simulink model "SENSORES"  (R2017b)
settings: Solver=FixedStepAuto  StartTime=0.0  StopTime=4.25  FixedStep=0.01  RelTol=1e-3  EnableMultiTasking=on
libraries: arduinolib x3
settings Model: SimulationMode=external  ExtModeTrigDuration=2  Creator=ferca  LastModifiedBy=Dr. Candia
settings OptimizationCC: EnhancedBackFolding=on  PassReuseOutputArgsThreshold=0  MaxStackSize=64  OptimizeBlockOrder=speed  DifferentSizesBufferReuse=on
settings DebuggingCC: ParameterTunabilityLossMsg=error
settings HardwareCC: ProdBitPerInt=16  ProdBitPerPointer=16  ProdBitPerSizeT=16  ProdBitPerPtrDiffT=16  ProdLargestAtomicFloat=None  ProdWordSize=8  ProdHWDeviceType=Atmel->AVR
settings SFSimCC: SimUseLocalCustomCode=on  MATLABDynamicMemAlloc=off
settings RTWCC: SystemTargetFile=ert.tlc  HardwareBoard=Arduino Uno  TLCOptions=-aInlineSetEventsForThisBaseRateFcn=TLC_FALSE -aSuppressMultiTaskScheduler=TLC_FALSE -aRateBasedStepFcn=1  TemplateMakefile=ert_default_tmf  GenerateReport=on  RTWUseLocalCustomCode=on  Toolchain=Arduino AVR  BuildConfiguration=Faster Runs  LaunchReport=on
settings CodeAppCC: ForceParamTrailComments=on  OperatorAnnotations=on  MangleLength=10
settings ERTTargetCC: ERTCustomFileBanners=off  SupportContinuousTime=on  SupportNonInlinedSFcns=on  RemoveResetFunc=off  SupportVariableSizeSignals=on  ModelStepFunctionPrototypeControlCompliant=off  ExtModeStaticAllocSize=2048

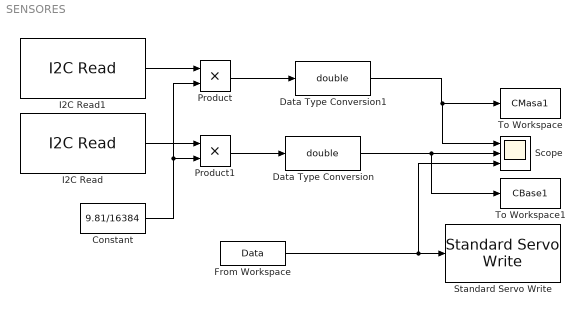
== system SENSORES ==
  Constant : Constant  Value=9.81/16384
  Data Type Conversion : DataTypeConversion  OutDataTypeStr=double
  Data Type Conversion1 : DataTypeConversion  OutDataTypeStr=double
  From Workspace : FromWorkspace  VariableName=Data  SampleTime=0.01  OutputAfterFinalValue=Holding final value
  I2C Read : arduinolib/I2C Read  SlaveAddress_=hex2dec( '69' )  RegisterAddressEnable=on  RegisterAddress_=hex2dec( '3C')  Datatype=uint16  ByteOrder=Big Endian  Datalength_=1  SampleTime_=0.01  blockPlatform=arduino
      settings: SourceProductName=Simulink Support Package for Arduino Hardware  SourceProductBaseCode=ARDUINO
  I2C Read1 : arduinolib/I2C Read  SlaveAddress_=hex2dec( '68' )  RegisterAddressEnable=on  RegisterAddress_=hex2dec( '3C' )  Datatype=uint16  ByteOrder=Big Endian  Datalength_=1  SampleTime_=0.01  blockPlatform=arduino
      settings: SourceProductName=Simulink Support Package for Arduino Hardware  SourceProductBaseCode=ARDUINO
  Product : Product
  Product1 : Product
  Scope : Scope  NumInputPorts=3
  Standard Servo Write : arduinolib/Standard Servo Write  pinNumber=9  blockPlatform=ARDUINO
      settings: SourceProductName=Simulink Support Package for Arduino Hardware
  To Workspace : ToWorkspace  VariableName=CMasa1  SaveFormat=Structure With Time  SampleTime=-1
      settings: Save2DSignal=2-D array (concatenate along first dimension)
  To Workspace1 : ToWorkspace  VariableName=CBase1  SaveFormat=Structure With Time  SampleTime=-1
      settings: Save2DSignal=2-D array (concatenate along first dimension)
  wires:
  Data Type Conversion/1 -> To Workspace1/1, Scope/2
  Data Type Conversion1/1 -> Scope/1, To Workspace/1
  Product/1 -> Data Type Conversion1/1
  Product1/1 -> Data Type Conversion/1
  Constant/1 -> Product/2, Product1/2
  I2C Read1/1 -> Product/1
  I2C Read/1 -> Product1/1
  From Workspace/1 -> Scope/3, Standard Servo Write/1
